simulink model "CDMA"  (R2022b)
settings: Solver=ode23s  StartTime=0.0  StopTime=0.0001  RelTol=1e-3
libraries: commsink2 x2, commdigbbndpm3 x2
settings Model: Creator=PMLS  LastModifiedBy=PMLS
settings DataIOCC: LoggingToFile=on

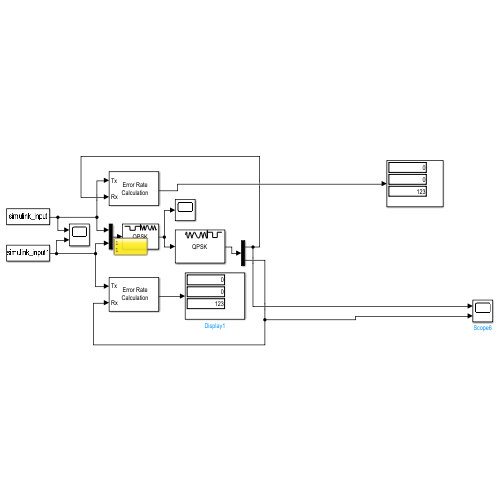
[thumbnail: Simulink's stored preview of the top-level diagram]
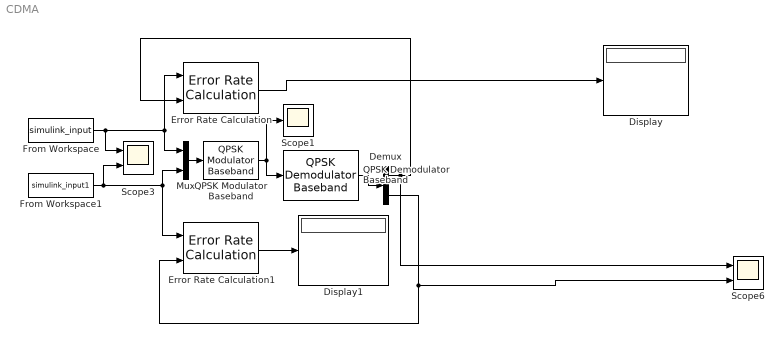
== system CDMA ==
  Demux : Demux  Outputs=2
  Display : Display
  Display1 : Display
  Error Rate Calculation : commsink2/Error Rate Calculation  N=0  st_delay=0  cp_mode=Entire frame  subframe=[]  PMode=Port  WsName=ErrorVec  RsMode2=off  stop=off  numErr=100  maxBits=1e6
  Error Rate Calculation1 : commsink2/Error Rate Calculation  N=0  st_delay=0  cp_mode=Entire frame  subframe=[]  PMode=Port  WsName=ErrorVec  RsMode2=off  stop=off  numErr=100  maxBits=1e6
  From Workspace : FromWorkspace  SampleTime=8.138020833333334e-07
  From Workspace1 : FromWorkspace  VariableName=simulink_input1  SampleTime=8.138020833333334e-07
  Mux : Mux  Inputs=2
  QPSK Demodulator Baseband : commdigbbndpm3/QPSK Demodulator Baseband  OutType=Bit  DecType=Hard decision  VarSource=Dialog  Variance=1  Dec=Binary  Ph=pi/4  outDtype1=Inherit via internal rule  outDtype2=Inherit via internal rule  derotateFactorWordLen=16  derotateFactorDataTypeStr=Inherit: Same word length as input  derotateFactorLastDataTypeStr=Inherit: Same word length as input
  QPSK Modulator Baseband : commdigbbndpm3/QPSK Modulator Baseband  InType=Bit  Enc=Binary  Ph=pi/4  outDtype=double  outWordLen=16  outUDDataType=sfix(16)  outFracLenMode=Best precision  outFracLen=15  outDataTypeStr=double  outLastDataTypeStr=double
      settings: LibrarySourceBlock=|
      | commhdldigbbndpm/QPSK
      | Modulator
      | Baseband
  Scope1 : Scope
  Scope3 : Scope  NumInputPorts=2
  Scope6 : Scope  NumInputPorts=2
  wires:
  Mux/1 -> QPSK Modulator Baseband/1
  From Workspace1/1 -> Mux/2, Error Rate Calculation1/1, Scope3/2
  From Workspace/1 -> Mux/1, Error Rate Calculation/1, Scope3/1
  QPSK Demodulator Baseband/1 -> Demux/1
  Demux/1 -> Scope6/1, Error Rate Calculation/2
  QPSK Modulator Baseband/1 -> Scope1/1, QPSK Demodulator Baseband/1
  Demux/2 -> Scope6/2, Error Rate Calculation1/2
  Error Rate Calculation1/1 -> Display1/1
  Error Rate Calculation/1 -> Display/1
